simulink model "MB_BOBShield_test"  (R2021b)
settings: Solver=FixedStepAuto  StartTime=0.0  StopTime=100  RelTol=1e-3  EnableMultiTasking=on
undefined symbols (not defined in the file or in its folder): Percentage
libraries: BOBShieldTest x3
settings Model: SimulationMode=external  ExtModeTrigDuration=2  Creator=micha  LastModifiedBy=micha
settings OptimizationCC: EnhancedBackFolding=on  PassReuseOutputArgsAs=Individual arguments  ZeroExternalMemoryAtStartup=off  ZeroInternalMemoryAtStartup=off  MaxStackSize=64  OptimizeBlockOrder=speed  DifferentSizesBufferReuse=on  OptimizationCustomize=off  EfficientTunableParamExpr=on
settings DebuggingCC: ParameterTunabilityLossMsg=error
settings HardwareCC: ProdBitPerInt=16  ProdBitPerPointer=16  ProdBitPerSizeT=16  ProdBitPerPtrDiffT=16  ProdLargestAtomicFloat=None  ProdWordSize=8  ProdHWDeviceType=Atmel->AVR
settings SFSimCC: MATLABDynamicMemAlloc=off
settings RTWCC: Description=Embedded Coder  SystemTargetFile=ert.tlc  HardwareBoard=Arduino Mega 2560  TemplateMakefile=ert_default_tmf  Toolchain=Arduino AVR  BuildConfiguration=Faster Runs
settings CodeAppCC: ForceParamTrailComments=on  IgnoreCustomStorageClasses=off  OperatorAnnotations=on  SimulinkDataObjDesc=on  SFDataObjDesc=on  InsertBlockDesc=on
settings ERTTargetCC: SupportContinuousTime=on  SupportVariableSizeSignals=on  ExtMode=on  ExtModeStaticAlloc=on  ExtModeStaticAllocSize=2048  ExtModeMexArgs='' 0 17725

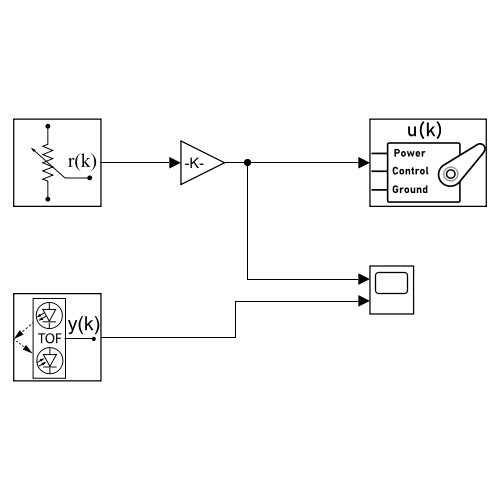
[thumbnail: Simulink's stored preview of the top-level diagram]
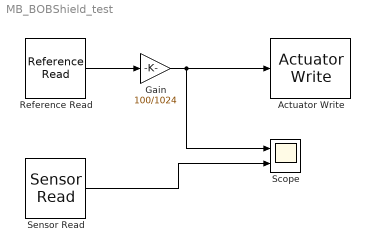
== system MB_BOBShield_test ==
  Actuator Write : BOBShieldTest/Actuator Write  InputType=Percentage (%)  RangeType=Default values (recommended)  MinAngle=-30  MaxAngle=30  Ts=0.025
      settings: SourceProductName=AutomationShield
  Gain : Gain  Gain=100/1024
  Reference Read : BOBShieldTest/Reference Read  ReadoutRadio=Analog value (ADC)  Ts=0.025
      settings: SourceProductName=AutomationShield
  Scope : Scope  NumInputPorts=2
  Sensor Read : BOBShieldTest/Sensor Read  OutRadio=Distance (mm)  CalType=Manual values  MinVal=5  MaxVal=100  Ts=0.025
      settings: SourceProductName=AutomationShield
  wires:
  Reference Read/1 -> Gain/1
  Gain/1 -> Scope/1, Actuator Write/1
  Sensor Read/1 -> Scope/2
